simulink model "observer_unit_test"  (R2015a)
settings: Solver=ode45  StartTime=0.0  StopTime=10  RelTol=1e-3
libraries: simulink x2
settings Model: Creator=MCLab  LastModifiedBy=MCLab

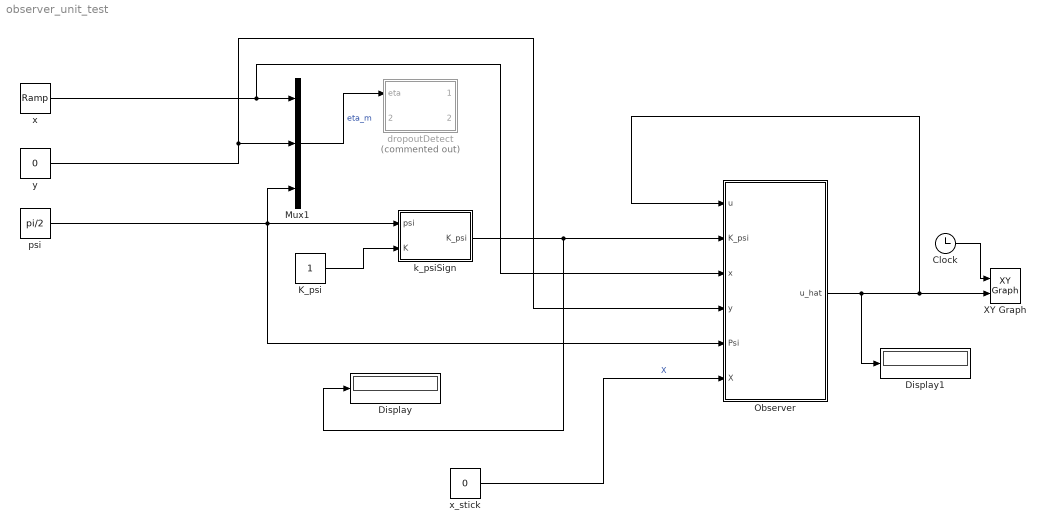
== system observer_unit_test ==
  Clock : Clock
  Display : Display
  Display1 : Display
  K_psi : Constant
  Mux1 : Mux  Inputs=3
  Observer : Subsystem
  XY Graph : simulink/Sinks/XY Graph  xmin=0  xmax=10  ymin=-.08  ymax=.08  st=-1
  dropoutDetect : MATLAB Function  Commented=on  TreatAsAtomicUnit=on
  k_psiSign : MATLAB Function  TreatAsAtomicUnit=on
  psi : Constant  Value=pi/2
  x : simulink/Sources/Ramp  slope=.05  start=0.2  X0=0
  "x_stick " : Constant  Value=0
  y : Constant  Value=0
  wires:
  x/1 -> Mux1/1, Observer/3(x)
  y/1 -> Observer/4("y "), Mux1/2
  psi/1 -> Observer/5(Psi), Mux1/3, k_psiSign/1(psi)
  "x_stick "/1 -> Observer/6(X)  "X"
  k_psiSign/1(K_psi) -> Display/1, Observer/2(K_psi)
  K_psi/1 -> k_psiSign/2(K)
  Mux1/1 -> dropoutDetect/1(eta)  "eta_m"
  Clock/1 -> XY Graph/1
  Observer/1(u_hat) -> Display1/1, XY Graph/2, Observer/1(u)

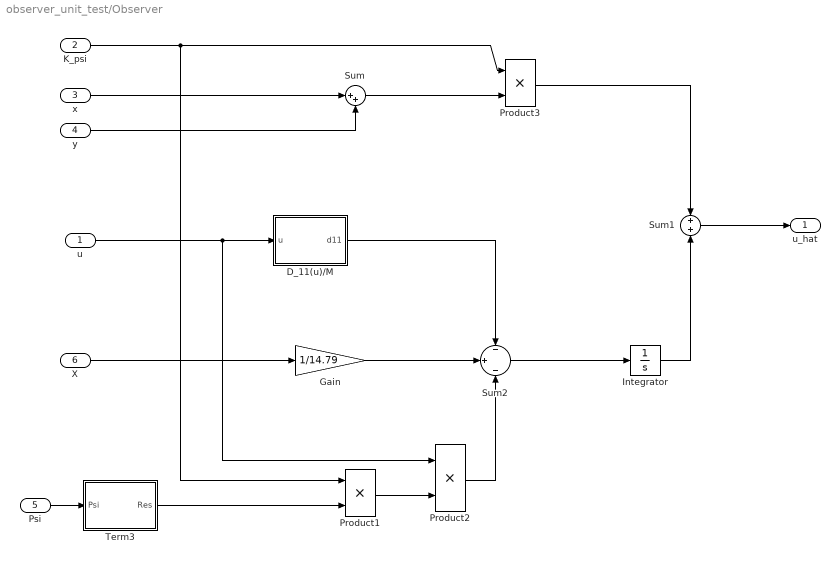
== system observer_unit_test/Observer ==
  u : Inport
  K_psi : Inport  Port=2
  x : Inport  Port=3
  "y " : Inport  Port=4
  Psi : Inport  Port=5
  X : Inport  Port=6
  D_11(u)/M : MATLAB Function  TreatAsAtomicUnit=on
  Gain : Gain  Gain=1/14.79
  Integrator : Integrator
  Product1 : Product
  Product2 : Product
  Product3 : Product
  Sum : Sum  Inputs=|++
  Sum1 : Sum  Inputs=+|+
  Sum2 : Sum  Inputs=-|+|-
  Term3 : MATLAB Function  TreatAsAtomicUnit=on
  u_hat : Outport
  wires:
  x/1 -> Sum/1
  K_psi/1 -> Product3/1, Product1/1
  Sum1/1 -> u_hat/1
  Sum2/1 -> Integrator/1
  Integrator/1 -> Sum1/2
  "y "/1 -> Sum/2
  u/1 -> Product2/1, D_11(u)/M/1(u)
  D_11(u)/M/1(d11) -> Sum2/1
  X/1 -> Gain/1
  Gain/1 -> Sum2/2
  Psi/1 -> Term3/1(Psi)
  Term3/1(Res) -> Product1/2
  Product1/1 -> Product2/2
  Product2/1 -> Sum2/3
  Product3/1 -> Sum1/1
  Sum/1 -> Product3/2

== matlab function observer_unit_test/k_psiSign ==
  data: psi input; K input; K_psi output
function K_psi = fcn(psi,K)

K_psi=K*sign(cos(psi)+sin(psi));


end

== matlab function observer_unit_test/Observer/D_11(u)//M ==
  data: u input; d11 output
function d11 = fcn(u)
%#codegen
%y = u;
d11=(0.6555-0.3545*abs(u)+3.787*u^2)*u/14.79;
end

== matlab function observer_unit_test/Observer/Term3 ==
  data: Psi input; Res output
function Res = fcn(Psi)

Res=cos(Psi)+sin(Psi);

end

== matlab function observer_unit_test/dropoutDetect ==
  data: eta input; dropout output; etaPrev input; etaOut output
function [dropout,etaOut]= fcn(eta,etaPrev)




end
